simulink model "Capstone_project_4"  (R2023a)
settings: Solver=VariableStepAuto  StartTime=0.0  StopTime=simtime  MaxStep=0.001  RelTol=1e-3
values from neighbouring files (symbols this model uses):
  b_1 = 1    [Capstone_project_4_workspace.mat]
  b_2 = 1    [Capstone_project_4_workspace.mat]
  F_in = 1    [Capstone_project_4_workspace.mat]
  k_1 = 1    [Capstone_project_4_workspace.mat]
  k_2 = 1    [Capstone_project_4_workspace.mat]
  m_1 = 1    [Capstone_project_4_workspace.mat]
  m_2 = 1    [Capstone_project_4_workspace.mat]
libraries: fl_lib x12, nesl_utility x6
settings Model: Creator=fycce  LastModifiedBy=fycce
settings DataIOCC: SaveOutput=off  SaveTime=off  ReturnWorkspaceOutputs=off

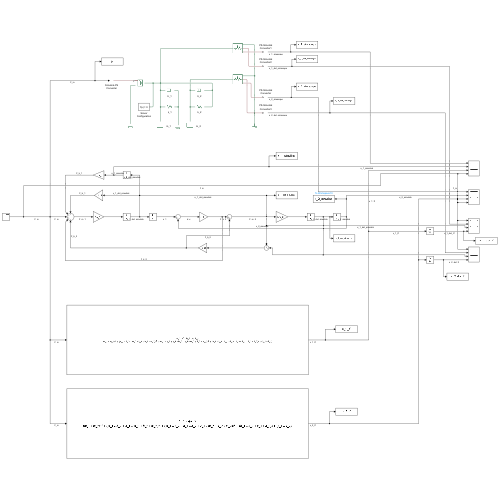
[thumbnail: Simulink's stored preview of the top-level diagram]
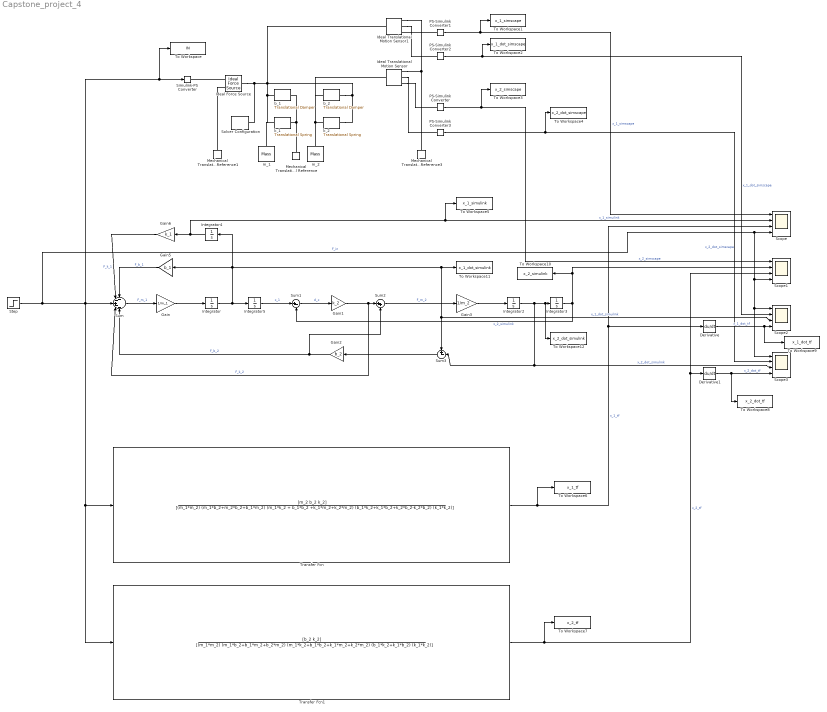
== system Capstone_project_4 ==
  Derivative : Derivative
  Derivative1 : Derivative
  Gain : Gain  Gain=1/m_1
  Gain1 : Gain  Gain=k_2
  Gain2 : Gain  Gain=b_2
  Gain3 : Gain  Gain=1/m_2
  Gain5 : Gain  Gain=b_1
  Gain6 : Gain  Gain=k_1
  Ideal Force Source : fl_lib/Mechanical/Mechanical Sources/Ideal Force Source
  Ideal Translational Motion Sensor : fl_lib/Mechanical/Mechanical Sensors/Ideal Translational Motion Sensor  reference=foundation.enum.MeasurementReference.difference  acceleration_port=false  velocity_port=true  position_port=true  offset=0 m
  Ideal Translational Motion Sensor1 : fl_lib/Mechanical/Mechanical Sensors/Ideal Translational Motion Sensor  reference=foundation.enum.MeasurementReference.difference  acceleration_port=false  velocity_port=true  position_port=true  offset=0 m
  Integrator{,2..5} (5 alike) : Integrator
  Mechanical Translational Reference : fl_lib/Mechanical/Translational Elements/Mechanical Translational Reference
  Mechanical Translational Reference1 : fl_lib/Mechanical/Translational Elements/Mechanical Translational Reference
  Mechanical Translational Reference3 : fl_lib/Mechanical/Translational Elements/Mechanical Translational Reference
  PS-Simulink Converter{,1..3} (4 alike) : nesl_utility/PS-Simulink Converter  PhysicalDomain=network_engine_domain  SubClassName=ps_output  LeftPortType=input  RightPortType=output  PseudoPeriodic=off  Frequencies=[]  VectorFormat=inherit  Unit=inherit  AffineConversion=off
  Scope{,1..3} (4 alike) : Scope  NumInputPorts=4
  Simulink-PS Converter : nesl_utility/Simulink-PS Converter  PhysicalDomain=network_engine_domain  SubClassName=ps_input  LeftPortType=input  RightPortType=output  PseudoPeriodic=off  Frequencies=[]  NoiseDistribution=none  NoiseParameters=[]  Unit=1  AffineConversion=off  FilteringAndDerivatives=provide  SimscapeFilterOrder=1  InputFilterTimeConstant=0.001  UdotUserProvided=0
  Solver Configuration : nesl_utility/Solver Configuration  PhysicalDomain=network_engine_domain  SubClassName=solver  LeftPortType=input  RightPortType=generic  Tones=[]  Harmonics=[]  SimulateNoise=off  Profile=off  UseLocalSampling=off  EnableSwitchedLinearOptims=on  FrequencyDomain=off  UseCCode=off  RelTol=0.001  AbsTol=1e-06  MinStep=1e-09  ToWorkspace=off  RevertToSquareIcSolve=off  NumHomotopyIterations=100  PhasorMode=off  PhasorModeNumHarmonics=1  ConsistencySolver=NEWTON_XTOL_AFTER_FTOL  IndexReductionMethod=DerivativeReplacement  DoDC=off  ResidualTolerance=1e-09  ConsistencyTolSource=GLOBAL  ConsistencyAbsTol=0.001  ConsistencyRelTol=0.001  ConsistencyTolFactor=0.001  UseLocalSolver=off  LocalSolverChoice=NE_BACKWARD_EULER_ADVANCER  ResolveIndetEquations=on  FunctionEvalNumThread=1  LocalSolverSampleTime=0.001  DoFixedCost=off  MaxNonlinIter=3  MaxModeIter=2  ComputeImpulses=off  ImpulseIterations=2  LinearAlgebra=auto  LinearAlgebraNumThread=0  EquationFormulation=NE_TIME_EF  DelaysMemoryBudget=1024  AutomaticFiltering=on  FilteringTimeConstant=0.001  PartitionStorageMethod=AS_NEEDED  PartitionMemoryBudget=1024  PartitionMethod=ROBUST
  Step : Step  After=F_in  SampleTime=0
  Sum : Sum  Inputs=--+--
  Sum1 : Sum  Inputs=|+-
  Sum2 : Sum  Inputs=|++
  Sum3 : Sum  Inputs=+-|
  To Workspace : ToWorkspace  VariableName=IN  SaveFormat=Timeseries  SampleTime=-1
  To Workspace1 : ToWorkspace  VariableName=x_1_simscape  SaveFormat=Timeseries  SampleTime=-1
  To Workspace10 : ToWorkspace  VariableName=x_2_simulink  SaveFormat=Timeseries  SampleTime=-1
  To Workspace11 : ToWorkspace  VariableName=x_1_dot_simulink  SaveFormat=Timeseries  SampleTime=-1
  To Workspace12 : ToWorkspace  VariableName=x_2_dot_simulink  SaveFormat=Timeseries  SampleTime=-1
  To Workspace2 : ToWorkspace  VariableName=x_1_dot_simscape  SaveFormat=Timeseries  SampleTime=-1
  To Workspace3 : ToWorkspace  VariableName=x_2_simscape  SaveFormat=Timeseries  SampleTime=-1
  To Workspace4 : ToWorkspace  VariableName=x_2_dot_simscape  SaveFormat=Timeseries  SampleTime=-1
  To Workspace5 : ToWorkspace  VariableName=x_1_simulink  SaveFormat=Timeseries  SampleTime=-1
  To Workspace6 : ToWorkspace  VariableName=x_1_tf  SaveFormat=Timeseries  SampleTime=-1
  To Workspace7 : ToWorkspace  VariableName=x_2_tf  SaveFormat=Timeseries  SampleTime=-1
  To Workspace8 : ToWorkspace  VariableName=x_2_dot_tf  SaveFormat=Timeseries  SampleTime=-1
  To Workspace9 : ToWorkspace  VariableName=x_1_dot_tf  SaveFormat=Timeseries  SampleTime=-1
  Transfer Fcn : TransferFcn  Numerator=[m_2 b_2 k_2]  Denominator=[(m_1*m_2) (m_1*b_2+m_2*b_2+b_1*m_2) (m_1*k_2 + b_1*b_2 +k_1*m_2+k_2*m_2) (b_1*k_2+k_1*b_2+k_2*b_2-k_2*b_2) (k_1*k_2)]
  Transfer Fcn1 : TransferFcn  Numerator=[b_2 k_2]  Denominator=[(m_1*m_2) (m_1*b_2+b_1*m_2+b_2*m_2) (m_1*k_2+b_1*b_2+k_1*m_2+k_2*m_2) (b_1*k_2+k_1*b_2) (k_1*k_2)]
  b_1 : fl_lib/Mechanical/Translational Elements/Translational Damper  D=b_1 N*s/m  v_specify=off  v_priority=None  v=0 m/s  v_nominal_specify=off  v_nominal_unit=m/s  v_nominal_value=1  f_specify=off  f_priority=None  f=0 N  f_nominal_specify=off  f_nominal_unit=N  f_nominal_value=1
  b_2 : fl_lib/Mechanical/Translational Elements/Translational Damper  D=b_2 N*s/m  v_specify=off  v_priority=None  v=0 m/s  v_nominal_specify=off  v_nominal_unit=m/s  v_nominal_value=1  f_specify=off  f_priority=None  f=0 N  f_nominal_specify=off  f_nominal_unit=N  f_nominal_value=1
  k_1 : fl_lib/Mechanical/Translational Elements/Translational Spring  spr_rate=k_1 N/m  v_specify=off  v_priority=None  v=0 m/s  v_nominal_specify=off  v_nominal_unit=m/s  v_nominal_value=1  f_specify=off  f_priority=None  f=0 N  f_nominal_specify=off  f_nominal_unit=N  f_nominal_value=1  x_specify=off  x_priority=High  x=0 m  x_nominal_specify=off  x_nominal_unit=m  x_nominal_value=1
  k_2 : fl_lib/Mechanical/Translational Elements/Translational Spring  spr_rate=k_2 N/m  v_specify=off  v_priority=None  v=0 m/s  v_nominal_specify=off  v_nominal_unit=m/s  v_nominal_value=1  f_specify=off  f_priority=None  f=0 N  f_nominal_specify=off  f_nominal_unit=N  f_nominal_value=1  x_specify=off  x_priority=High  x=0 m  x_nominal_specify=off  x_nominal_unit=m  x_nominal_value=1
  m_1 : fl_lib/Mechanical/Translational Elements/Mass  mass=m_1 kg  num_ports=foundation.enum.numPorts2.one  v_specify=off  v_priority=High  v=0 m/s  v_nominal_specify=off  v_nominal_unit=m/s  v_nominal_value=1  f_specify=off  f_priority=None  f=0 N  f_nominal_specify=off  f_nominal_unit=N  f_nominal_value=1
  m_2 : fl_lib/Mechanical/Translational Elements/Mass  mass=m_2 kg  num_ports=foundation.enum.numPorts2.one  v_specify=off  v_priority=High  v=0 m/s  v_nominal_specify=off  v_nominal_unit=m/s  v_nominal_value=1  f_specify=off  f_priority=None  f=0 N  f_nominal_specify=off  f_nominal_unit=N  f_nominal_value=1
  wires:
  Gain5/1 -> Sum/1  "F_b_1"
  Gain2/1 -> Sum2/2, Sum/5  "F_b_2"
  Integrator4/1 -> To Workspace5/1, Scope/2, Gain6/1  "x_1_simulink"
  Gain6/1 -> Sum/2  "F_k_1"
  Sum3/1 -> Gain2/1
  Sum1/1 -> Gain1/1  "d_x"
  Gain/1 -> Integrator/1
  Integrator/1 -> Integrator5/1, Sum3/1, Scope2/3, To Workspace11/1, Integrator4/1, Gain5/1  "x_1_dot_simulink"
  Gain1/1 -> Sum2/1, Sum/4  "F_k_2"
  Integrator5/1 -> Sum1/1  "x_1"
  Sum/1 -> Gain/1  "F_m_1"
  Gain3/1 -> Integrator2/1
  Step/1 -> Scope1/4, Scope2/1, Scope3/1, Scope/4, To Workspace/1, Simulink-PS Converter/1, Sum/3, Transfer Fcn1/1, Transfer Fcn/1  "F_in"
  Integrator3/1 -> To Workspace10/1, Scope1/2, Sum1/2  "x_2_simulink"
  Sum2/1 -> Gain3/1  "F_m_2"
  Integrator2/1 -> Scope3/3, Sum3/2, To Workspace12/1, Integrator3/1  "x_2_dot_simulink"
  PS-Simulink Converter1/1 -> To Workspace1/1, Scope/1  "x_1_simscape"
  Transfer Fcn/1 -> To Workspace6/1, Scope/3, Derivative/1  "x_1_tf"
  PS-Simulink Converter/1 -> To Workspace3/1, Scope1/1  "x_2_simscape"
  Transfer Fcn1/1 -> To Workspace7/1, Derivative1/1, Scope1/3  "x_2_tf"
  Derivative/1 -> Scope2/4, To Workspace9/1  "x_1_dot_tf"
  Derivative1/1 -> To Workspace8/1, Scope3/4  "x_2_dot_tf"
  PS-Simulink Converter2/1 -> To Workspace2/1, Scope2/2  "x_1_dot_simscape"
  PS-Simulink Converter3/1 -> To Workspace4/1, Scope3/2  "x_2_dot_simscape"
  connections:
  Ideal Force Source/LConn1 -- Solver Configuration/RConn1 -- k_2/RConn1 -- b_2/RConn1 -- Ideal Translational Motion Sensor1/LConn1 -- k_1/LConn1 -- m_1/LConn1 -- b_1/LConn1
  Ideal Translational Motion Sensor1/RConn1 -- Mechanical Translational Reference3/LConn1 -- Ideal Translational Motion Sensor/RConn1
  PS-Simulink Converter1/LConn1 -- Ideal Translational Motion Sensor1/RConn3
  Ideal Force Source/RConn2 -- Mechanical Translational Reference1/LConn1
  Ideal Translational Motion Sensor/RConn3 -- PS-Simulink Converter/LConn1
  Ideal Force Source/RConn1 -- Simulink-PS Converter/RConn1
  m_2/LConn1 -- Ideal Translational Motion Sensor/LConn1 -- b_2/LConn1 -- k_2/LConn1
  k_1/RConn1 -- Mechanical Translational Reference/LConn1 -- b_1/RConn1
  Ideal Translational Motion Sensor1/RConn2 -- PS-Simulink Converter2/LConn1
  Ideal Translational Motion Sensor/RConn2 -- PS-Simulink Converter3/LConn1
